simulink model "simplified_powertrain"  (R2020b)
settings: Solver=FixedStepAuto  StartTime=0.0  StopTime=60  RelTol=1e-3
PreLoadFcn:
  | C_sc = 1;
StartFcn:
  | C_sc = 1;
values from neighbouring files (symbols this model uses):
  D = 0    [model_fc.m]
undefined symbols (not defined in the file or in its folder): command, DiscIntNeverNeededParam, ECMS, Flight, in, Ion, Lithium, out, w
libraries: powerlib x22, electricdrivelib x3, lib_converters x3, simulink x2, fuzblock x1, mpclib x1, re_lib x1
(part 2 of 6)

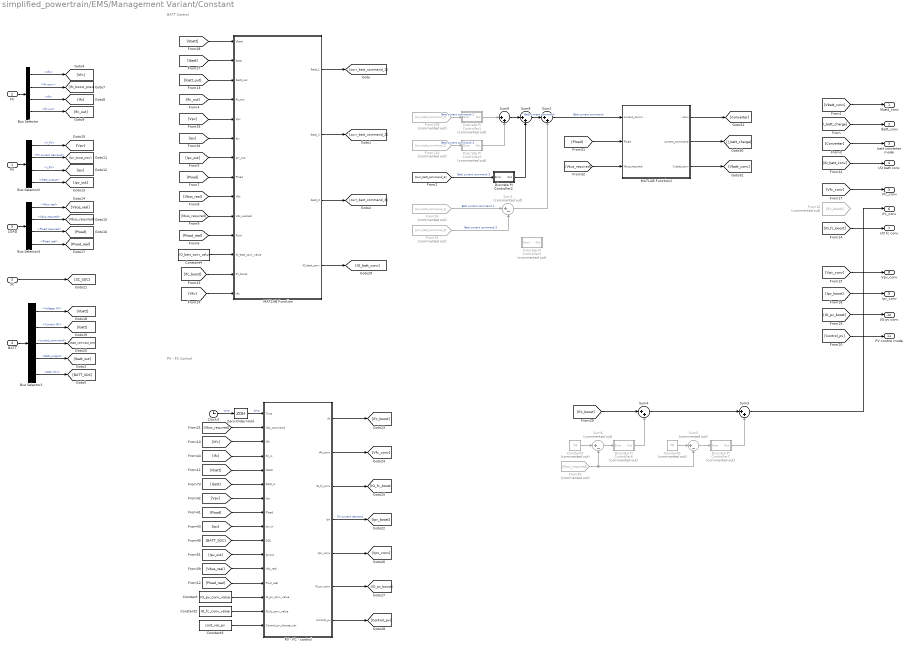
== system simplified_powertrain/EMS/Management Variant/Constant ==
  note: BATT Control
  note: PV - FC Control
  PV : Inport
  FC : Inport  Port=2
  SC : Inport  Port=3
  BATT : Inport  Port=4
  LOAD : Inport  Port=5
  Bus Selector : BusSelector  OutputSignals=Vfc,Ifc conv,Ifc,Ifc out
  Bus Selector1 : BusSelector  OutputSignals=Voltage (V),Current (A),current_command,Ibatt_output,SOC (%)
  Bus Selector2 : BusSelector  OutputSignals=V_PV,PV current demand,I_PV,Ibatt_output
  Bus Selector3 : BusSelector  OutputSignals=Vbus real,Vbus required,Pload required,Pload real
  Clock3 : Clock
  Constant : Constant  Value=IO_pv_conv_value
  Constant2 : Constant  Value=IO_fc_conv_value
  Constant3 : Constant  Value=cont_var_pv
  Constant4 : Constant  Value=IO_batt_conv_value
  Constant5 : Constant  Commented=on  Value=74
  Constant6 : Constant  Commented=on  Value=70
  Discrete PI Controller1 : Subsystem  Commented=on  DialogController=POWERSYS.PowerSysDialog  mask(Discrete PI Controller){Kp=1, Ki=10, Par_Limits=[100 -100], Init=0, Ts=1e-4}
      mask prompts: Kp "Proportional gain (Kp):"; Ki "Integral gain (Ki):"; Par_Limits "Output limits: [ Upper   Lower ]"; Init "Output initial value:"; Ts "Sample time:"
      mask help: This block implements a discrete PI controller.
      mask init:
      | UpperLimit=Par_Limits(1);
      | LowerLimit=Par_Limits(2);
      | power_initmask();
      mask Help: This block is part of a subset of blocks in the Extras library that does not have documentation associated with it, other than the block mask description.
      mask Display: disp('PI');
  Discrete PI Controller2 : Subsystem  DialogController=POWERSYS.PowerSysDialog  mask(Discrete PI Controller){Kp=10, Ki=100, Par_Limits=[100 -100], Init=0, Ts=1e-4}
      mask prompts: Kp "Proportional gain (Kp):"; Ki "Integral gain (Ki):"; Par_Limits "Output limits: [ Upper   Lower ]"; Init "Output initial value:"; Ts "Sample time:"
      mask help: This block implements a discrete PI controller.
      mask init:
      | UpperLimit=Par_Limits(1);
      | LowerLimit=Par_Limits(2);
      | power_initmask();
      mask Help: This block is part of a subset of blocks in the Extras library that does not have documentation associated with it, other than the block mask description.
      mask Display: disp('PI');
  Discrete PI Controller3 : Subsystem  Commented=on  DialogController=POWERSYS.PowerSysDialog  mask(Discrete PI Controller){Kp=10, Ki=1, Par_Limits=[100 -100], Init=0, Ts=1e-4}
      mask prompts: Kp "Proportional gain (Kp):"; Ki "Integral gain (Ki):"; Par_Limits "Output limits: [ Upper   Lower ]"; Init "Output initial value:"; Ts "Sample time:"
      mask help: This block implements a discrete PI controller.
      mask init:
      | UpperLimit=Par_Limits(1);
      | LowerLimit=Par_Limits(2);
      | power_initmask();
      mask Help: This block is part of a subset of blocks in the Extras library that does not have documentation associated with it, other than the block mask description.
      mask Display: disp('PI');
  Discrete PI Controller5 : Subsystem  Commented=on  DialogController=POWERSYS.PowerSysDialog  mask(Discrete PI Controller){Kp=10, Ki=10, Par_Limits=[50 -20], Init=0, Ts=1e-4}
      mask prompts: Kp "Proportional gain (Kp):"; Ki "Integral gain (Ki):"; Par_Limits "Output limits: [ Upper   Lower ]"; Init "Output initial value:"; Ts "Sample time:"
      mask help: This block implements a discrete PI controller.
      mask init:
      | UpperLimit=Par_Limits(1);
      | LowerLimit=Par_Limits(2);
      | power_initmask();
      mask Help: This block is part of a subset of blocks in the Extras library that does not have documentation associated with it, other than the block mask description.
      mask Display: disp('PI');
  Discrete PI Controller6 : Subsystem  Commented=on  DialogController=POWERSYS.PowerSysDialog  mask(Discrete PI Controller){Kp=10, Ki=10, Par_Limits=[40 0], Init=0, Ts=1e-4}
      mask prompts: Kp "Proportional gain (Kp):"; Ki "Integral gain (Ki):"; Par_Limits "Output limits: [ Upper   Lower ]"; Init "Output initial value:"; Ts "Sample time:"
      mask help: This block implements a discrete PI controller.
      mask init:
      | UpperLimit=Par_Limits(1);
      | LowerLimit=Par_Limits(2);
      | power_initmask();
      mask Help: This block is part of a subset of blocks in the Extras library that does not have documentation associated with it, other than the block mask description.
      mask Display: disp('PI');
  Discrete PI Controller7 : Subsystem  Commented=on  DialogController=POWERSYS.PowerSysDialog  mask(Discrete PI Controller){Kp=10, Ki=10, Par_Limits=[0 -40], Init=0, Ts=1e-4}
      mask prompts: Kp "Proportional gain (Kp):"; Ki "Integral gain (Ki):"; Par_Limits "Output limits: [ Upper   Lower ]"; Init "Output initial value:"; Ts "Sample time:"
      mask help: This block implements a discrete PI controller.
      mask init:
      | UpperLimit=Par_Limits(1);
      | LowerLimit=Par_Limits(2);
      | power_initmask();
      mask Help: This block is part of a subset of blocks in the Extras library that does not have documentation associated with it, other than the block mask description.
      mask Display: disp('PI');
  From108 : From  Commented=on  GotoTag=curr_batt_command_1
  From110 : From  Commented=on  GotoTag=curr_batt_command_2
  From16 : From  Commented=on  GotoTag=Ifc_boost
  From25 : From  Commented=on  GotoTag=curr_batt_command_3
  From26 : From  Commented=on  GotoTag=curr_batt_command_1
  From30 : From  Commented=on  GotoTag=Vbus_required
  MATLAB Function : MATLAB Function  TreatAsAtomicUnit=on
  MATLAB Function1 : MATLAB Function  TreatAsAtomicUnit=on
  PV - FC - control : MATLAB Function  TreatAsAtomicUnit=on
  Sum1 : Sum  Commented=on  Inputs=|+-
  Sum{2..4,8..9} (5 alike) : Sum  Inputs=|++
  Sum5 : Sum  Commented=on  Inputs=|+-
  Sum6 : Sum  Commented=on  Inputs=|+-
  Zero-Order Hold : ZeroOrderHold  SampleTime=1e-4
  Vbatt_conv : Outport
  Ibatt_conv : Outport  Port=2
  batt converter mode : Outport  Port=3
  I/O batt conv : Outport  Port=4
  Vfc_conv : Outport  Port=5
  Ifc_conv : Outport  Port=6
  I/O fc conv : Outport  Port=7
  Vpv_conv : Outport  Port=8
  Ipv_conv : Outport  Port=9
  I/O pv conv : Outport  Port=10
  PV control mode : Outport  Port=11
  wires:
  Constant/1 -> PV - FC - control/14(IO_pv_conv_value)
  MATLAB Function1/1(conv) -> [Converter]
  [Vbatt] -> MATLAB Function/1(Vbatt)
  [Ibatt_out] -> MATLAB Function/3(Ibatt_out)
  Bus Selector1/5 -> [BATT_SOC]  "<SOC (%)>"
  From30/1 -> Sum5/2, Sum6/2
  [Vpv] -> MATLAB Function/5(Vpv)
  Sum6/1 -> Discrete PI Controller6/1(Error)
  Discrete PI Controller7/1(Out) -> Sum3/2
  PV - FC - control/3(IO_fc_conv) -> [IO_fc_boost]
  [Ifc_out] -> MATLAB Function/4(Ifc_out)
  Bus Selector1/3 -> [Ibatt_command_pre]  "<current_command>"
  [IO_fc_boost] -> I/O fc conv/1
  MATLAB Function1/3(V_batt_conv) -> [Vbatt_conv]
  Bus Selector1/2 -> [Ibatt]  "<Current (A)>"
  [Ifc_boost] -> MATLAB Function/13(Ifc_boost)
  [Vbus_required] -> MATLAB Function1/3(Vbus_required)
  Sum2/1 -> MATLAB Function1/1(current_comm)  "Batt current command"
  [Vpv_conv] -> Vpv_conv/1
  Bus Selector1/1 -> [Vbatt]  "<Voltage (V)>"
  [Ibatt] -> PV - FC - control/6(Ibatt_in)
  From26/1 -> Sum1/1  "Batt current command 1"
  Bus Selector1/4 -> [Ibatt_out]  "<Ibatt_output>"
  MATLAB Function1/2(current_command) -> [I_batt_charge]
  [Ipv_boost] -> Ipv_conv/1
  [Pload_real] -> MATLAB Function/11(Pout)
  PV - FC - control/5(Vpv_conv) -> [Vpv_conv]
  Constant6/1 -> Sum5/1
  Sum5/1 -> Discrete PI Controller7/1(Error)
  Constant2/1 -> PV - FC - control/15(IO_fc_conv_value)
  MATLAB Function/2(Ibatt_2) -> [curr_batt_command_2]
  MATLAB Function/1(Ibatt_1) -> [curr_batt_command_1]
  Bus Selector2/1 -> [Vpv]  "<V_PV>"
  [Pload] -> MATLAB Function1/2(Pload)
  Sum4/1 -> Sum3/1
  [Ifc_boost] -> Sum4/1
  From25/1 -> Sum1/2  "Batt current command 3"
  [Ibatt] -> MATLAB Function/2(Ibatt)
  [IO_pv_boost] -> I/O pv conv/1
  [Vfc] -> MATLAB Function/14(Vfc)
  Bus Selector2/3 -> [Ipv]  "<I_PV>"
  Sum1/1 -> Sum2/2
  [Vfc_conv] -> Vfc_conv/1
  [Ipv_out] -> PV - FC - control/11(Ipvout)
  PV - FC - control/7(Control_pv) -> [Control_pv]
  [Vbus_required] -> PV - FC - control/2(Vdc_command)
  [Vbatt_conv] -> Vbatt_conv/1
  [Vbus_real] -> PV - FC - control/12(Vdc_real)
  MATLAB Function/4(IO_batt_conv) -> [IO_batt_conv]
  Constant3/1 -> PV - FC - control/16(Control_pv_choose_var)
  PV - FC - control/1(Ifc) -> [Ifc_boost]
  FC/1 -> Bus Selector/1
  [Ipv] -> PV - FC - control/9(Ipv_in)
  Sum8/1 -> Sum2/1  "Batt current command"
  Zero-Order Hold/1 -> PV - FC - control/1(Time)  "time"
  [Pload] -> MATLAB Function/8(Pload)
  [Vbus_required] -> MATLAB Function/10(Vdc_wanted)
  Clock3/1 -> Zero-Order Hold/1  "time"
  [Pload_real] -> PV - FC - control/13(Pout_real)
  [Vpv] -> PV - FC - control/7(Vpv)
  LOAD/1 -> Bus Selector3/1
  Constant5/1 -> Sum6/1
  [Control_pv] -> PV control mode/1
  Bus Selector/3 -> [Ifc]  "<Ifc>"
  [Ipv_out] -> MATLAB Function/7(Ipv_out)
  From110/1 -> Discrete PI Controller3/1(Error)  "Batt current command 3"
  [IO_batt_conv] -> I/O batt conv/1
  [Vbus_real] -> MATLAB Function/9(Vdc)
  Bus Selector3/3 -> [Pload]  "<Pload required>"
  Bus Selector2/4 -> [Ipv_out]  "<Ibatt_output>"
  PV - FC - control/4(Ipv) -> [Ipv_boost]  "PV current demand"
  [Ifc] -> PV - FC - control/4(Ifc_in)
  Bus Selector3/2 -> [Vbus_required]  "<Vbus required>"
  BATT/1 -> Bus Selector1/1
  Discrete PI Controller6/1(Out) -> Sum4/2
  Bus Selector2/2 -> [Ipv_boost_prev]  "<PV current demand>"
  Bus Selector3/1 -> [Vbus_real]  "<Vbus real>"
  Constant4/1 -> MATLAB Function/12(IO_batt_conv_value)
  PV - FC - control/6(IO_pv_conv) -> [IO_pv_boost]
  SC/1 -> [SC_SOC]
  [Converter] -> batt converter mode/1
  PV - FC - control/2(Vfc_conv) -> [Vfc_conv]
  [I_batt_charge] -> Ibatt_conv/1
  [Vbatt] -> PV - FC - control/5(Vbatt)
  [Vfc] -> PV - FC - control/3(Vfc)
  [curr_batt_command_3] -> Discrete PI Controller2/1(Error)  "Batt current command 3"
  Bus Selector/1 -> [Vfc]  "<Vfc>"
  Bus Selector/4 -> [Ifc_out]  "<Ifc out>"
  PV/1 -> Bus Selector2/1
  [Pload] -> PV - FC - control/8(Pload)
  Bus Selector/2 -> [Ifc_boost_prev]  "<Ifc conv>"
  Sum9/1 -> Sum8/1
  From108/1 -> Discrete PI Controller1/1(Error)  "Batt current command 1"
  Discrete PI Controller2/1(Out) -> Sum8/2
  MATLAB Function/3(Ibatt_3) -> [curr_batt_command_3]
  Sum3/1 -> Ifc_conv/1
  Discrete PI Controller1/1(Out) -> Sum9/1
  Discrete PI Controller3/1(Out) -> Sum9/2
  [BATT_SOC] -> PV - FC - control/10(SOC)
  [Ipv] -> MATLAB Function/6(Ipv)
  Bus Selector3/4 -> [Pload_real]  "<Pload real>"

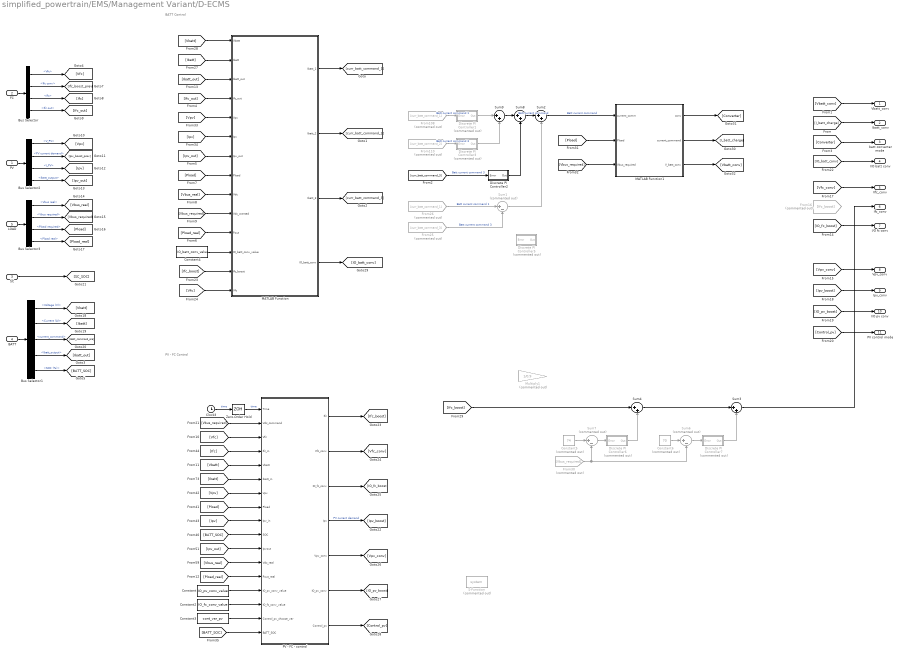
== system simplified_powertrain/EMS/Management Variant/D-ECMS ==
  note: PV - FC Control
  note: BATT Control
  PV : Inport
  FC : Inport  Port=2
  SC : Inport  Port=3
  BATT : Inport  Port=4
  LOAD : Inport  Port=5
  Bus Selector : BusSelector  OutputSignals=Vfc,Ifc conv,Ifc,Ifc out
  Bus Selector1 : BusSelector  OutputSignals=Voltage (V),Current (A),current_command,Ibatt_output,SOC (%)
  Bus Selector2 : BusSelector  OutputSignals=V_PV,PV current demand,I_PV,Ibatt_output
  Bus Selector3 : BusSelector  OutputSignals=Vbus real,Vbus required,Pload required,Pload real
  Clock3 : Clock
  Constant : Constant  Value=IO_pv_conv_value
  Constant2 : Constant  Value=IO_fc_conv_value
  Constant3 : Constant  Value=cont_var_pv
  Constant4 : Constant  Value=IO_batt_conv_value
  Constant5 : Constant  Commented=on  Value=74
  Constant6 : Constant  Commented=on  Value=70
  Discrete PI Controller1 : Subsystem  Commented=on  DialogController=POWERSYS.PowerSysDialog  mask(Discrete PI Controller){Kp=1, Ki=10, Par_Limits=[100 -100], Init=0, Ts=1e-4}
      mask prompts: Kp "Proportional gain (Kp):"; Ki "Integral gain (Ki):"; Par_Limits "Output limits: [ Upper   Lower ]"; Init "Output initial value:"; Ts "Sample time:"
      mask help: This block implements a discrete PI controller.
      mask init:
      | UpperLimit=Par_Limits(1);
      | LowerLimit=Par_Limits(2);
      | power_initmask();
      mask Help: This block is part of a subset of blocks in the Extras library that does not have documentation associated with it, other than the block mask description.
      mask Display: disp('PI');
  Discrete PI Controller2 : Subsystem  DialogController=POWERSYS.PowerSysDialog  mask(Discrete PI Controller){Kp=10, Ki=100, Par_Limits=[50 -20], Init=0, Ts=1e-4}
      mask prompts: Kp "Proportional gain (Kp):"; Ki "Integral gain (Ki):"; Par_Limits "Output limits: [ Upper   Lower ]"; Init "Output initial value:"; Ts "Sample time:"
      mask help: This block implements a discrete PI controller.
      mask init:
      | UpperLimit=Par_Limits(1);
      | LowerLimit=Par_Limits(2);
      | power_initmask();
      mask Help: This block is part of a subset of blocks in the Extras library that does not have documentation associated with it, other than the block mask description.
      mask Display: disp('PI');
  Discrete PI Controller3 : Subsystem  Commented=on  DialogController=POWERSYS.PowerSysDialog  mask(Discrete PI Controller){Kp=10, Ki=1, Par_Limits=[100 -100], Init=0, Ts=1e-4}
      mask prompts: Kp "Proportional gain (Kp):"; Ki "Integral gain (Ki):"; Par_Limits "Output limits: [ Upper   Lower ]"; Init "Output initial value:"; Ts "Sample time:"
      mask help: This block implements a discrete PI controller.
      mask init:
      | UpperLimit=Par_Limits(1);
      | LowerLimit=Par_Limits(2);
      | power_initmask();
      mask Help: This block is part of a subset of blocks in the Extras library that does not have documentation associated with it, other than the block mask description.
      mask Display: disp('PI');
  Discrete PI Controller5 : Subsystem  Commented=on  DialogController=POWERSYS.PowerSysDialog  mask(Discrete PI Controller){Kp=10, Ki=10, Par_Limits=[50 -20], Init=0, Ts=1e-4}
      mask prompts: Kp "Proportional gain (Kp):"; Ki "Integral gain (Ki):"; Par_Limits "Output limits: [ Upper   Lower ]"; Init "Output initial value:"; Ts "Sample time:"
      mask help: This block implements a discrete PI controller.
      mask init:
      | UpperLimit=Par_Limits(1);
      | LowerLimit=Par_Limits(2);
      | power_initmask();
      mask Help: This block is part of a subset of blocks in the Extras library that does not have documentation associated with it, other than the block mask description.
      mask Display: disp('PI');
  Discrete PI Controller6 : Subsystem  Commented=on  DialogController=POWERSYS.PowerSysDialog  mask(Discrete PI Controller){Kp=10, Ki=10, Par_Limits=[40 0], Init=0, Ts=1e-4}
      mask prompts: Kp "Proportional gain (Kp):"; Ki "Integral gain (Ki):"; Par_Limits "Output limits: [ Upper   Lower ]"; Init "Output initial value:"; Ts "Sample time:"
      mask help: This block implements a discrete PI controller.
      mask init:
      | UpperLimit=Par_Limits(1);
      | LowerLimit=Par_Limits(2);
      | power_initmask();
      mask Help: This block is part of a subset of blocks in the Extras library that does not have documentation associated with it, other than the block mask description.
      mask Display: disp('PI');
  Discrete PI Controller7 : Subsystem  Commented=on  DialogController=POWERSYS.PowerSysDialog  mask(Discrete PI Controller){Kp=10, Ki=10, Par_Limits=[0 -40], Init=0, Ts=1e-4}
      mask prompts: Kp "Proportional gain (Kp):"; Ki "Integral gain (Ki):"; Par_Limits "Output limits: [ Upper   Lower ]"; Init "Output initial value:"; Ts "Sample time:"
      mask help: This block implements a discrete PI controller.
      mask init:
      | UpperLimit=Par_Limits(1);
      | LowerLimit=Par_Limits(2);
      | power_initmask();
      mask Help: This block is part of a subset of blocks in the Extras library that does not have documentation associated with it, other than the block mask description.
      mask Display: disp('PI');
  From108 : From  Commented=on  GotoTag=curr_batt_command_1
  From110 : From  Commented=on  GotoTag=curr_batt_command_2
  From16 : From  Commented=on  GotoTag=Ifc_boost
  From25 : From  Commented=on  GotoTag=curr_batt_command_3
  From26 : From  Commented=on  GotoTag=curr_batt_command_1
  From30 : From  Commented=on  GotoTag=Vbus_required
  MATLAB Function : MATLAB Function  TreatAsAtomicUnit=on
  MATLAB Function1 : MATLAB Function  TreatAsAtomicUnit=on
  Multiply1 : Gain  Commented=on  Gain=1/0.9
  PV - FC - control : MATLAB Function  TreatAsAtomicUnit=on
  S-Function : S-Function  Commented=on  SFunctionDeploymentMode=off  EnableBusSupport=off
  Sum1 : Sum  Commented=on  Inputs=|+-
  Sum{2..4,8..9} (5 alike) : Sum  Inputs=|++
  Sum6 : Sum  Commented=on  Inputs=|+-
  Sum7 : Sum  Commented=on  Inputs=|+-
  Zero-Order Hold : ZeroOrderHold  SampleTime=1e-4
  Vbatt_conv : Outport
  Ibatt_conv : Outport  Port=2
  batt converter mode : Outport  Port=3
  I/O batt conv : Outport  Port=4
  Vfc_conv : Outport  Port=5
  Ifc_conv : Outport  Port=6
  I/O fc conv : Outport  Port=7
  Vpv_conv : Outport  Port=8
  Ipv_conv : Outport  Port=9
  I/O pv conv : Outport  Port=10
  PV control mode : Outport  Port=11
  wires:
  [Ipv_out] -> PV - FC - control/11(Ipvout)
  Sum1/1 -> Sum2/2
  PV - FC - control/7(Control_pv) -> [Control_pv]
  [Vbus_required] -> PV - FC - control/2(Vdc_command)
  MATLAB Function/4(IO_batt_conv) -> [IO_batt_conv]
  Constant3/1 -> PV - FC - control/16(Control_pv_choose_var)
  [Vbatt_conv] -> Vbatt_conv/1
  [Vbus_real] -> PV - FC - control/12(Vdc_real)
  [Pload] -> MATLAB Function/8(Pload)
  Zero-Order Hold/1 -> PV - FC - control/1(Time)  "time"
  [Ipv] -> PV - FC - control/9(Ipv_in)
  Sum8/1 -> Sum2/1  "Batt current command"
  [Vpv] -> PV - FC - control/7(Vpv)
  LOAD/1 -> Bus Selector3/1
  Clock3/1 -> Zero-Order Hold/1  "time"
  [Control_pv] -> PV control mode/1
  [Ipv_out] -> MATLAB Function/7(Ipv_out)
  Bus Selector/3 -> [Ifc]  "<Ifc>"
  [IO_batt_conv] -> I/O batt conv/1
  Bus Selector3/3 -> [Pload]  "<Pload required>"
  PV - FC - control/4(Ipv) -> [Ipv_boost]  "PV current demand"
  Bus Selector2/4 -> [Ipv_out]  "<Ibatt_output>"
  [Ifc_boost] -> Sum4/1
  [Vbus_required] -> MATLAB Function/10(Vdc_wanted)
  [BATT_SOC] -> PV - FC - control/17(BATT_SOC)
  PV/1 -> Bus Selector2/1
  [curr_batt_command_3] -> Discrete PI Controller2/1(Error)  "Batt current command 3"
  From110/1 -> Discrete PI Controller3/1(Error)  "Batt current command 3"
  [Vbus_required] -> MATLAB Function1/3(Vbus_required)
  Bus Selector1/3 -> [Ibatt_command_pre]  "<current_command>"
  PV - FC - control/3(IO_fc_conv) -> [IO_fc_boost]
  [Ifc_out] -> MATLAB Function/4(Ifc_out)
  [Vpv_conv] -> Vpv_conv/1
  Bus Selector1/2 -> [Ibatt]  "<Current (A)>"
  MATLAB Function1/3(V_batt_conv) -> [Vbatt_conv]
  [Ifc_boost] -> MATLAB Function/13(Ifc_boost)
  Bus Selector/2 -> [Ifc_boost_prev]  "<Ifc conv>"
  Bus Selector3/4 -> [Pload_real]  "<Pload real>"
  Discrete PI Controller3/1(Out) -> Sum9/2
  [Ifc] -> PV - FC - control/4(Ifc_in)
  Discrete PI Controller6/1(Out) -> Sum4/2
  [Vbatt] -> MATLAB Function/1(Vbatt)
  PV - FC - control/6(IO_pv_conv) -> [IO_pv_boost]
  Discrete PI Controller2/1(Out) -> Sum8/2
  Bus Selector1/5 -> [BATT_SOC]  "<SOC (%)>"
  Bus Selector1/4 -> [Ibatt_out]  "<Ibatt_output>"
  [Vbatt] -> PV - FC - control/5(Vbatt)
  [Ipv_boost] -> Ipv_conv/1
  Sum7/1 -> Discrete PI Controller6/1(Error)
  Bus Selector3/2 -> [Vbus_required]  "<Vbus required>"
  Bus Selector3/1 -> [Vbus_real]  "<Vbus real>"
  Bus Selector2/2 -> [Ipv_boost_prev]  "<PV current demand>"
  FC/1 -> Bus Selector/1
  PV - FC - control/2(Vfc_conv) -> [Vfc_conv]
  Bus Selector/4 -> [Ifc_out]  "<Ifc out>"
  PV - FC - control/1(Ifc) -> [Ifc_boost]
  [BATT_SOC] -> PV - FC - control/10(SOC)
  [Vfc] -> PV - FC - control/3(Vfc)
  [Pload] -> PV - FC - control/8(Pload)
  Sum6/1 -> Discrete PI Controller7/1(Error)
  From26/1 -> Sum1/1  "Batt current command 1"
  [Pload_real] -> MATLAB Function/11(Pout)
  PV - FC - control/5(Vpv_conv) -> [Vpv_conv]
  MATLAB Function1/2(current_command) -> [I_batt_charge]
  [Ibatt_out] -> MATLAB Function/3(Ibatt_out)
  Constant6/1 -> Sum6/1
  Sum4/1 -> Sum3/1
  SC/1 -> [SC_SOC]
  [Ipv] -> MATLAB Function/6(Ipv)
  Bus Selector2/1 -> [Vpv]  "<V_PV>"
  Constant2/1 -> PV - FC - control/15(IO_fc_conv_value)
  [Pload] -> MATLAB Function1/2(Pload)
  MATLAB Function/1(Ibatt_1) -> [curr_batt_command_1]
  Constant5/1 -> Sum7/1
  Constant4/1 -> MATLAB Function/12(IO_batt_conv_value)
  MATLAB Function/2(Ibatt_2) -> [curr_batt_command_2]
  [IO_fc_boost] -> I/O fc conv/1
  [Ibatt] -> MATLAB Function/2(Ibatt)
  From108/1 -> Discrete PI Controller1/1(Error)  "Batt current command 1"
  [IO_pv_boost] -> I/O pv conv/1
  Bus Selector2/3 -> [Ipv]  "<I_PV>"
  [Vfc] -> MATLAB Function/14(Vfc)
  MATLAB Function/3(Ibatt_3) -> [curr_batt_command_3]
  From25/1 -> Sum1/2  "Batt current command 3"
  BATT/1 -> Bus Selector1/1
  Sum3/1 -> Ifc_conv/1
  [Vfc_conv] -> Vfc_conv/1
  Sum2/1 -> MATLAB Function1/1(current_comm)  "Batt current command"
  Bus Selector/1 -> [Vfc]  "<Vfc>"
  [Pload_real] -> PV - FC - control/13(Pout_real)
  [Ibatt] -> PV - FC - control/6(Ibatt_in)
  [Vpv] -> MATLAB Function/5(Vpv)
  [Vbus_real] -> MATLAB Function/9(Vdc)
  Discrete PI Controller7/1(Out) -> Sum3/2
  Bus Selector1/1 -> [Vbatt]  "<Voltage (V)>"
  Sum9/1 -> Sum8/1
  [Converter] -> batt converter mode/1
  MATLAB Function1/1(conv) -> [Converter]
  Constant/1 -> PV - FC - control/14(IO_pv_conv_value)
  [I_batt_charge] -> Ibatt_conv/1
  From30/1 -> Sum6/2, Sum7/2
  Discrete PI Controller1/1(Out) -> Sum9/1

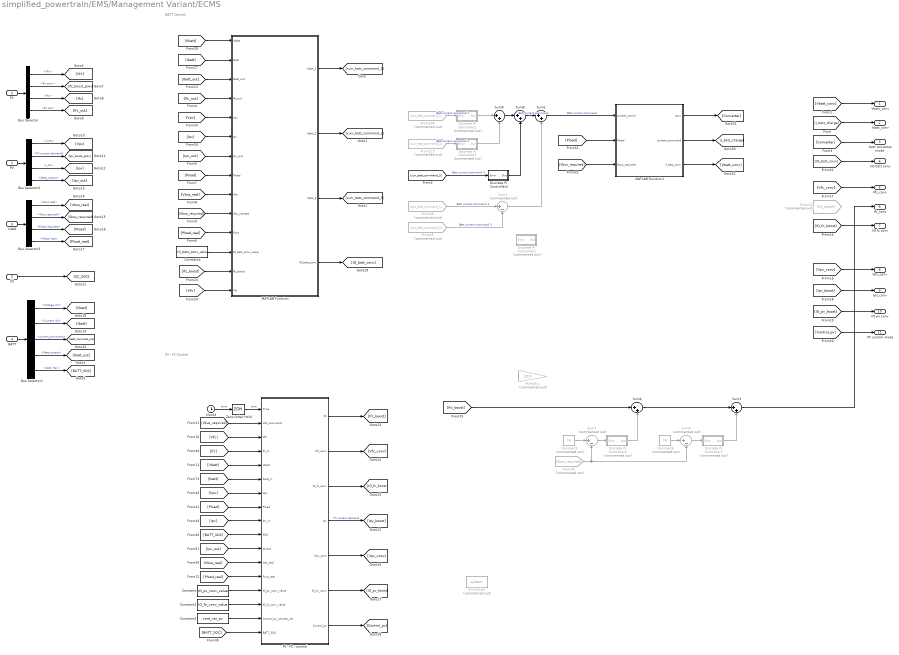
== system simplified_powertrain/EMS/Management Variant/ECMS ==
  note: PV - FC Control
  note: BATT Control
  PV : Inport
  FC : Inport  Port=2
  SC : Inport  Port=3
  BATT : Inport  Port=4
  LOAD : Inport  Port=5
  Bus Selector : BusSelector  OutputSignals=Vfc,Ifc conv,Ifc,Ifc out
  Bus Selector1 : BusSelector  OutputSignals=Voltage (V),Current (A),current_command,Ibatt_output,SOC (%)
  Bus Selector2 : BusSelector  OutputSignals=V_PV,PV current demand,I_PV,Ibatt_output
  Bus Selector3 : BusSelector  OutputSignals=Vbus real,Vbus required,Pload required,Pload real
  Clock3 : Clock
  Constant : Constant  Value=IO_pv_conv_value
  Constant2 : Constant  Value=IO_fc_conv_value
  Constant3 : Constant  Value=cont_var_pv
  Constant4 : Constant  Value=IO_batt_conv_value
  Constant5 : Constant  Commented=on  Value=74
  Constant6 : Constant  Commented=on  Value=70
  Discrete PI Controller1 : Subsystem  Commented=on  DialogController=POWERSYS.PowerSysDialog  mask(Discrete PI Controller){Kp=1, Ki=10, Par_Limits=[100 -100], Init=0, Ts=1e-4}
      mask prompts: Kp "Proportional gain (Kp):"; Ki "Integral gain (Ki):"; Par_Limits "Output limits: [ Upper   Lower ]"; Init "Output initial value:"; Ts "Sample time:"
      mask help: This block implements a discrete PI controller.
      mask init:
      | UpperLimit=Par_Limits(1);
      | LowerLimit=Par_Limits(2);
      | power_initmask();
      mask Help: This block is part of a subset of blocks in the Extras library that does not have documentation associated with it, other than the block mask description.
      mask Display: disp('PI');
  Discrete PI Controller2 : Subsystem  DialogController=POWERSYS.PowerSysDialog  mask(Discrete PI Controller){Kp=10, Ki=100, Par_Limits=[50 -20], Init=0, Ts=1e-4}
      mask prompts: Kp "Proportional gain (Kp):"; Ki "Integral gain (Ki):"; Par_Limits "Output limits: [ Upper   Lower ]"; Init "Output initial value:"; Ts "Sample time:"
      mask help: This block implements a discrete PI controller.
      mask init:
      | UpperLimit=Par_Limits(1);
      | LowerLimit=Par_Limits(2);
      | power_initmask();
      mask Help: This block is part of a subset of blocks in the Extras library that does not have documentation associated with it, other than the block mask description.
      mask Display: disp('PI');
  Discrete PI Controller3 : Subsystem  Commented=on  DialogController=POWERSYS.PowerSysDialog  mask(Discrete PI Controller){Kp=10, Ki=1, Par_Limits=[100 -100], Init=0, Ts=1e-4}
      mask prompts: Kp "Proportional gain (Kp):"; Ki "Integral gain (Ki):"; Par_Limits "Output limits: [ Upper   Lower ]"; Init "Output initial value:"; Ts "Sample time:"
      mask help: This block implements a discrete PI controller.
      mask init:
      | UpperLimit=Par_Limits(1);
      | LowerLimit=Par_Limits(2);
      | power_initmask();
      mask Help: This block is part of a subset of blocks in the Extras library that does not have documentation associated with it, other than the block mask description.
      mask Display: disp('PI');
  Discrete PI Controller5 : Subsystem  Commented=on  DialogController=POWERSYS.PowerSysDialog  mask(Discrete PI Controller){Kp=10, Ki=10, Par_Limits=[50 -20], Init=0, Ts=1e-4}
      mask prompts: Kp "Proportional gain (Kp):"; Ki "Integral gain (Ki):"; Par_Limits "Output limits: [ Upper   Lower ]"; Init "Output initial value:"; Ts "Sample time:"
      mask help: This block implements a discrete PI controller.
      mask init:
      | UpperLimit=Par_Limits(1);
      | LowerLimit=Par_Limits(2);
      | power_initmask();
      mask Help: This block is part of a subset of blocks in the Extras library that does not have documentation associated with it, other than the block mask description.
      mask Display: disp('PI');
  Discrete PI Controller6 : Subsystem  Commented=on  DialogController=POWERSYS.PowerSysDialog  mask(Discrete PI Controller){Kp=10, Ki=10, Par_Limits=[40 0], Init=0, Ts=1e-4}
      mask prompts: Kp "Proportional gain (Kp):"; Ki "Integral gain (Ki):"; Par_Limits "Output limits: [ Upper   Lower ]"; Init "Output initial value:"; Ts "Sample time:"
      mask help: This block implements a discrete PI controller.
      mask init:
      | UpperLimit=Par_Limits(1);
      | LowerLimit=Par_Limits(2);
      | power_initmask();
      mask Help: This block is part of a subset of blocks in the Extras library that does not have documentation associated with it, other than the block mask description.
      mask Display: disp('PI');
  Discrete PI Controller7 : Subsystem  Commented=on  DialogController=POWERSYS.PowerSysDialog  mask(Discrete PI Controller){Kp=10, Ki=10, Par_Limits=[0 -40], Init=0, Ts=1e-4}
      mask prompts: Kp "Proportional gain (Kp):"; Ki "Integral gain (Ki):"; Par_Limits "Output limits: [ Upper   Lower ]"; Init "Output initial value:"; Ts "Sample time:"
      mask help: This block implements a discrete PI controller.
      mask init:
      | UpperLimit=Par_Limits(1);
      | LowerLimit=Par_Limits(2);
      | power_initmask();
      mask Help: This block is part of a subset of blocks in the Extras library that does not have documentation associated with it, other than the block mask description.
      mask Display: disp('PI');
  From108 : From  Commented=on  GotoTag=curr_batt_command_1
  From110 : From  Commented=on  GotoTag=curr_batt_command_2
  From16 : From  Commented=on  GotoTag=Ifc_boost
  From25 : From  Commented=on  GotoTag=curr_batt_command_3
  From26 : From  Commented=on  GotoTag=curr_batt_command_1
  From30 : From  Commented=on  GotoTag=Vbus_required
  MATLAB Function : MATLAB Function  TreatAsAtomicUnit=on
  MATLAB Function1 : MATLAB Function  TreatAsAtomicUnit=on
  Multiply1 : Gain  Commented=on  Gain=1/0.9
  PV - FC - control : MATLAB Function  TreatAsAtomicUnit=on
  S-Function : S-Function  Commented=on  SFunctionDeploymentMode=off  EnableBusSupport=off
  Sum1 : Sum  Commented=on  Inputs=|+-
  Sum{2..4,8..9} (5 alike) : Sum  Inputs=|++
  Sum6 : Sum  Commented=on  Inputs=|+-
  Sum7 : Sum  Commented=on  Inputs=|+-
  Zero-Order Hold : ZeroOrderHold  SampleTime=1e-4
  Vbatt_conv : Outport
  Ibatt_conv : Outport  Port=2
  batt converter mode : Outport  Port=3
  I/O batt conv : Outport  Port=4
  Vfc_conv : Outport  Port=5
  Ifc_conv : Outport  Port=6
  I/O fc conv : Outport  Port=7
  Vpv_conv : Outport  Port=8
  Ipv_conv : Outport  Port=9
  I/O pv conv : Outport  Port=10
  PV control mode : Outport  Port=11
  wires:
  [Ipv_out] -> PV - FC - control/11(Ipvout)
  Sum1/1 -> Sum2/2
  PV - FC - control/7(Control_pv) -> [Control_pv]
  [Vbus_required] -> PV - FC - control/2(Vdc_command)
  MATLAB Function/4(IO_batt_conv) -> [IO_batt_conv]
  Constant3/1 -> PV - FC - control/16(Control_pv_choose_var)
  [Vbatt_conv] -> Vbatt_conv/1
  [Vbus_real] -> PV - FC - control/12(Vdc_real)
  [Pload] -> MATLAB Function/8(Pload)
  Zero-Order Hold/1 -> PV - FC - control/1(Time)  "time"
  [Ipv] -> PV - FC - control/9(Ipv_in)
  Sum8/1 -> Sum2/1  "Batt current command"
  [Vpv] -> PV - FC - control/7(Vpv)
  LOAD/1 -> Bus Selector3/1
  Clock3/1 -> Zero-Order Hold/1  "time"
  [Control_pv] -> PV control mode/1
  [Ipv_out] -> MATLAB Function/7(Ipv_out)
  Bus Selector/3 -> [Ifc]  "<Ifc>"
  [IO_batt_conv] -> I/O batt conv/1
  Bus Selector3/3 -> [Pload]  "<Pload required>"
  PV - FC - control/4(Ipv) -> [Ipv_boost]  "PV current demand"
  Bus Selector2/4 -> [Ipv_out]  "<Ibatt_output>"
  [Ifc_boost] -> Sum4/1
  [Vbus_required] -> MATLAB Function/10(Vdc_wanted)
  [BATT_SOC] -> PV - FC - control/17(BATT_SOC)
  PV/1 -> Bus Selector2/1
  [curr_batt_command_3] -> Discrete PI Controller2/1(Error)  "Batt current command 3"
  From110/1 -> Discrete PI Controller3/1(Error)  "Batt current command 3"
  [Vbus_required] -> MATLAB Function1/3(Vbus_required)
  Bus Selector1/3 -> [Ibatt_command_pre]  "<current_command>"
  PV - FC - control/3(IO_fc_conv) -> [IO_fc_boost]
  [Ifc_out] -> MATLAB Function/4(Ifc_out)
  [Vpv_conv] -> Vpv_conv/1
  Bus Selector1/2 -> [Ibatt]  "<Current (A)>"
  MATLAB Function1/3(V_batt_conv) -> [Vbatt_conv]
  [Ifc_boost] -> MATLAB Function/13(Ifc_boost)
  Bus Selector/2 -> [Ifc_boost_prev]  "<Ifc conv>"
  Bus Selector3/4 -> [Pload_real]  "<Pload real>"
  Discrete PI Controller3/1(Out) -> Sum9/2
  [Ifc] -> PV - FC - control/4(Ifc_in)
  Discrete PI Controller6/1(Out) -> Sum4/2
  [Vbatt] -> MATLAB Function/1(Vbatt)
  PV - FC - control/6(IO_pv_conv) -> [IO_pv_boost]
  Discrete PI Controller2/1(Out) -> Sum8/2
  Bus Selector1/5 -> [BATT_SOC]  "<SOC (%)>"
  Bus Selector1/4 -> [Ibatt_out]  "<Ibatt_output>"
  [Vbatt] -> PV - FC - control/5(Vbatt)
  [Ipv_boost] -> Ipv_conv/1
  Sum7/1 -> Discrete PI Controller6/1(Error)
  Bus Selector3/2 -> [Vbus_required]  "<Vbus required>"
  Bus Selector3/1 -> [Vbus_real]  "<Vbus real>"
  Bus Selector2/2 -> [Ipv_boost_prev]  "<PV current demand>"
  FC/1 -> Bus Selector/1
  PV - FC - control/2(Vfc_conv) -> [Vfc_conv]
  Bus Selector/4 -> [Ifc_out]  "<Ifc out>"
  PV - FC - control/1(Ifc) -> [Ifc_boost]
  [BATT_SOC] -> PV - FC - control/10(SOC)
  [Vfc] -> PV - FC - control/3(Vfc)
  [Pload] -> PV - FC - control/8(Pload)
  Sum6/1 -> Discrete PI Controller7/1(Error)
  From26/1 -> Sum1/1  "Batt current command 1"
  [Pload_real] -> MATLAB Function/11(Pout)
  PV - FC - control/5(Vpv_conv) -> [Vpv_conv]
  MATLAB Function1/2(current_command) -> [I_batt_charge]
  [Ibatt_out] -> MATLAB Function/3(Ibatt_out)
  Constant6/1 -> Sum6/1
  Sum4/1 -> Sum3/1
  SC/1 -> [SC_SOC]
  [Ipv] -> MATLAB Function/6(Ipv)
  Bus Selector2/1 -> [Vpv]  "<V_PV>"
  Constant2/1 -> PV - FC - control/15(IO_fc_conv_value)
  [Pload] -> MATLAB Function1/2(Pload)
  MATLAB Function/1(Ibatt_1) -> [curr_batt_command_1]
  Constant5/1 -> Sum7/1
  Constant4/1 -> MATLAB Function/12(IO_batt_conv_value)
  MATLAB Function/2(Ibatt_2) -> [curr_batt_command_2]
  [IO_fc_boost] -> I/O fc conv/1
  [Ibatt] -> MATLAB Function/2(Ibatt)
  From108/1 -> Discrete PI Controller1/1(Error)  "Batt current command 1"
  [IO_pv_boost] -> I/O pv conv/1
  Bus Selector2/3 -> [Ipv]  "<I_PV>"
  [Vfc] -> MATLAB Function/14(Vfc)
  MATLAB Function/3(Ibatt_3) -> [curr_batt_command_3]
  From25/1 -> Sum1/2  "Batt current command 3"
  BATT/1 -> Bus Selector1/1
  Sum3/1 -> Ifc_conv/1
  [Vfc_conv] -> Vfc_conv/1
  Sum2/1 -> MATLAB Function1/1(current_comm)  "Batt current command"
  Bus Selector/1 -> [Vfc]  "<Vfc>"
  [Pload_real] -> PV - FC - control/13(Pout_real)
  [Ibatt] -> PV - FC - control/6(Ibatt_in)
  [Vpv] -> MATLAB Function/5(Vpv)
  [Vbus_real] -> MATLAB Function/9(Vdc)
  Discrete PI Controller7/1(Out) -> Sum3/2
  Bus Selector1/1 -> [Vbatt]  "<Voltage (V)>"
  Sum9/1 -> Sum8/1
  [Converter] -> batt converter mode/1
  MATLAB Function1/1(conv) -> [Converter]
  Constant/1 -> PV - FC - control/14(IO_pv_conv_value)
  [I_batt_charge] -> Ibatt_conv/1
  From30/1 -> Sum6/2, Sum7/2
  Discrete PI Controller1/1(Out) -> Sum9/1

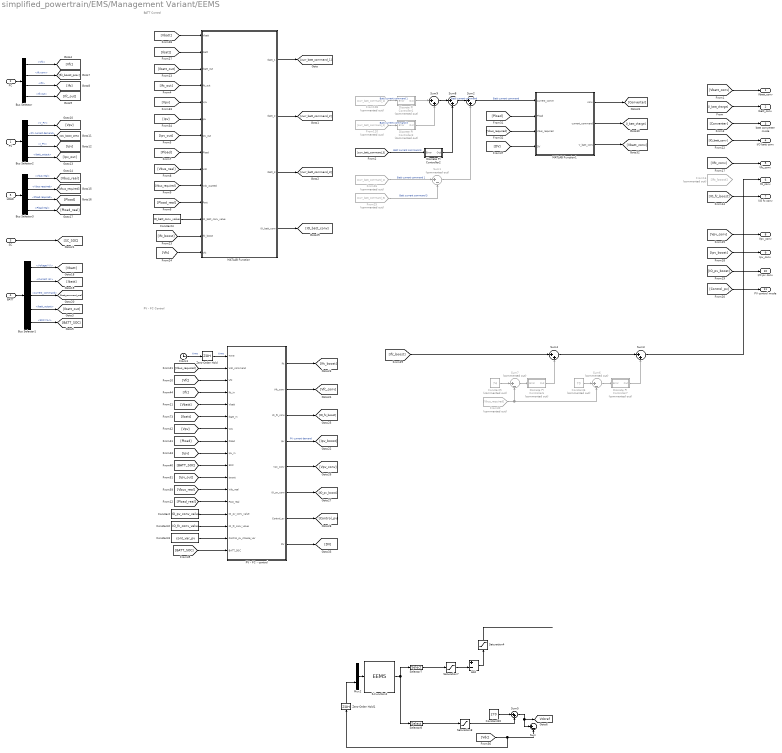
== system simplified_powertrain/EMS/Management Variant/EEMS ==
  note: PV - FC Control
  note: BATT Control
  PV : Inport
  FC : Inport  Port=2
  SC : Inport  Port=3
  BATT : Inport  Port=4
  LOAD : Inport  Port=5
  Add : Sum  Inputs=+-
  Bus Selector : BusSelector  OutputSignals=Vfc,Ifc conv,Ifc,Ifc out
  Bus Selector1 : BusSelector  OutputSignals=Voltage (V),Current (A),current_command,Ibatt_output,SOC (%)
  Bus Selector2 : BusSelector  OutputSignals=V_PV,PV current demand,I_PV,Ibatt_output
  Bus Selector3 : BusSelector  OutputSignals=Vbus real,Vbus required,Pload required,Pload real
  Clock3 : Clock
  Constant : Constant  Value=IO_pv_conv_value
  Constant2 : Constant  Value=IO_fc_conv_value
  Constant20 : Constant  Value=270
  Constant3 : Constant  Value=cont_var_pv
  Constant4 : Constant  Value=IO_batt_conv_value
  Constant5 : Constant  Commented=on  Value=74
  Constant6 : Constant  Commented=on  Value=70
  Discrete PI Controller1 : Subsystem  Commented=on  DialogController=POWERSYS.PowerSysDialog  mask(Discrete PI Controller){Kp=1, Ki=10, Par_Limits=[100 -100], Init=0, Ts=1e-4}
      mask prompts: Kp "Proportional gain (Kp):"; Ki "Integral gain (Ki):"; Par_Limits "Output limits: [ Upper   Lower ]"; Init "Output initial value:"; Ts "Sample time:"
      mask help: This block implements a discrete PI controller.
      mask init:
      | UpperLimit=Par_Limits(1);
      | LowerLimit=Par_Limits(2);
      | power_initmask();
      mask Help: This block is part of a subset of blocks in the Extras library that does not have documentation associated with it, other than the block mask description.
      mask Display: disp('PI');
  Discrete PI Controller2 : Subsystem  DialogController=POWERSYS.PowerSysDialog  mask(Discrete PI Controller){Kp=10, Ki=100, Par_Limits=[100 -100], Init=0, Ts=1e-4}
      mask prompts: Kp "Proportional gain (Kp):"; Ki "Integral gain (Ki):"; Par_Limits "Output limits: [ Upper   Lower ]"; Init "Output initial value:"; Ts "Sample time:"
      mask help: This block implements a discrete PI controller.
      mask init:
      | UpperLimit=Par_Limits(1);
      | LowerLimit=Par_Limits(2);
      | power_initmask();
      mask Help: This block is part of a subset of blocks in the Extras library that does not have documentation associated with it, other than the block mask description.
      mask Display: disp('PI');
  Discrete PI Controller3 : Subsystem  Commented=on  DialogController=POWERSYS.PowerSysDialog  mask(Discrete PI Controller){Kp=10, Ki=1, Par_Limits=[100 -100], Init=0, Ts=1e-4}
      mask prompts: Kp "Proportional gain (Kp):"; Ki "Integral gain (Ki):"; Par_Limits "Output limits: [ Upper   Lower ]"; Init "Output initial value:"; Ts "Sample time:"
      mask help: This block implements a discrete PI controller.
      mask init:
      | UpperLimit=Par_Limits(1);
      | LowerLimit=Par_Limits(2);
      | power_initmask();
      mask Help: This block is part of a subset of blocks in the Extras library that does not have documentation associated with it, other than the block mask description.
      mask Display: disp('PI');
  Discrete PI Controller6 : Subsystem  Commented=on  DialogController=POWERSYS.PowerSysDialog  mask(Discrete PI Controller){Kp=10, Ki=10, Par_Limits=[40 0], Init=0, Ts=1e-4}
      mask prompts: Kp "Proportional gain (Kp):"; Ki "Integral gain (Ki):"; Par_Limits "Output limits: [ Upper   Lower ]"; Init "Output initial value:"; Ts "Sample time:"
      mask help: This block implements a discrete PI controller.
      mask init:
      | UpperLimit=Par_Limits(1);
      | LowerLimit=Par_Limits(2);
      | power_initmask();
      mask Help: This block is part of a subset of blocks in the Extras library that does not have documentation associated with it, other than the block mask description.
      mask Display: disp('PI');
  Discrete PI Controller7 : Subsystem  Commented=on  DialogController=POWERSYS.PowerSysDialog  mask(Discrete PI Controller){Kp=10, Ki=10, Par_Limits=[0 -40], Init=0, Ts=1e-4}
      mask prompts: Kp "Proportional gain (Kp):"; Ki "Integral gain (Ki):"; Par_Limits "Output limits: [ Upper   Lower ]"; Init "Output initial value:"; Ts "Sample time:"
      mask help: This block implements a discrete PI controller.
      mask init:
      | UpperLimit=Par_Limits(1);
      | LowerLimit=Par_Limits(2);
      | power_initmask();
      mask Help: This block is part of a subset of blocks in the Extras library that does not have documentation associated with it, other than the block mask description.
      mask Display: disp('PI');
  From108 : From  Commented=on  GotoTag=curr_batt_command_1
  From110 : From  Commented=on  GotoTag=curr_batt_command_2
  From16 : From  Commented=on  GotoTag=Ifc_boost
  From25 : From  Commented=on  GotoTag=curr_batt_command_3
  From26 : From  Commented=on  GotoTag=curr_batt_command_1
  From30 : From  Commented=on  GotoTag=Vbus_required
  MATLAB Function : MATLAB Function  TreatAsAtomicUnit=on
  MATLAB Function1 : MATLAB Function  TreatAsAtomicUnit=on
  Mux2 : Mux  Inputs=2
  PV - FC - control : MATLAB Function  TreatAsAtomicUnit=on
  S-Function2 : S-Function  FunctionName=EEMS  SFunctionDeploymentMode=off  EnableBusSupport=off
  Saturation4 : Saturate  UpperLimit=8800  LowerLimit=850
  Saturation7 : Saturate  UpperLimit=3400  LowerLimit=-1500
  Saturation8 : Saturate  UpperLimit=2  LowerLimit=-2
  Selector7 : Selector  InputPortWidth=2  IndexOptions=Index vector (dialog)  Indices=1  OutputSizes=1
  Selector8 : Selector  InputPortWidth=2  IndexOptions=Index vector (dialog)  Indices=2  OutputSizes=1
  Sum : Sum  Inputs=|+-
  Sum1 : Sum  Commented=on  Inputs=|+-
  Sum{2..5,8..9} (6 alike) : Sum  Inputs=|++
  Sum6 : Sum  Commented=on  Inputs=|+-
  Sum7 : Sum  Commented=on  Inputs=|+-
  Zero-Order Hold : ZeroOrderHold  SampleTime=1e-4
  Zero-Order Hold1 : ZeroOrderHold  SampleTime=200e-3
  Vbatt_conv : Outport
  Ibatt_conv : Outport  Port=2
  batt converter mode : Outport  Port=3
  I/O batt conv : Outport  Port=4
  Vfc_conv : Outport  Port=5
  Ifc_conv : Outport  Port=6
  I/O fc conv : Outport  Port=7
  Vpv_conv : Outport  Port=8
  Ipv_conv : Outport  Port=9
  I/O pv conv : Outport  Port=10
  PV control mode : Outport  Port=11
  tag scope: Vdcref=global
  wires:
  [Ipv_out] -> PV - FC - control/11(Ipvout)
  Sum1/1 -> Sum2/2
  PV - FC - control/7(Control_pv) -> [Control_pv]
  [Vbus_required] -> PV - FC - control/2(Vdc_command)
  MATLAB Function/4(IO_batt_conv) -> [IO_batt_conv]
  Constant3/1 -> PV - FC - control/16(Control_pv_choose_var)
  [Vbatt_conv] -> Vbatt_conv/1
  [Vbus_real] -> PV - FC - control/12(Vdc_real)
  [Pload] -> MATLAB Function/8(Pload)
  Zero-Order Hold/1 -> PV - FC - control/1(Time)  "time"
  [Ipv] -> PV - FC - control/9(Ipv_in)
  Sum8/1 -> Sum2/1  "Batt current command"
  [Vpv] -> PV - FC - control/7(Vpv)
  LOAD/1 -> Bus Selector3/1
  Clock3/1 -> Zero-Order Hold/1  "time"
  [Control_pv] -> PV control mode/1
  [Ipv_out] -> MATLAB Function/7(Ipv_out)
  Bus Selector/3 -> [Ifc]  "<Ifc>"
  [IO_batt_conv] -> I/O batt conv/1
  Bus Selector3/3 -> [Pload]  "<Pload required>"
  PV - FC - control/4(Ipv) -> [Ipv_boost]  "PV current demand"
  Bus Selector2/4 -> [Ipv_out]  "<Ibatt_output>"
  [Ifc_boost] -> Sum4/1
  [Vbus_required] -> MATLAB Function/10(Vdc_wanted)
  [BATT_SOC] -> PV - FC - control/17(BATT_SOC)
  PV/1 -> Bus Selector2/1
  [curr_batt_command_3] -> Discrete PI Controller2/1(Error)  "Batt current command 3"
  From110/1 -> Discrete PI Controller3/1(Error)  "Batt current command 3"
  [Vbus_required] -> MATLAB Function1/3(Vbus_required)
  Bus Selector1/3 -> [Ibatt_command_pre]  "<current_command>"
  PV - FC - control/3(IO_fc_conv) -> [IO_fc_boost]
  [Ifc_out] -> MATLAB Function/4(Ifc_out)
  [Vpv_conv] -> Vpv_conv/1
  Bus Selector1/2 -> [Ibatt]  "<Current (A)>"
  MATLAB Function1/3(V_batt_conv) -> [Vbatt_conv]
  [Ifc_boost] -> MATLAB Function/13(Ifc_boost)
  Bus Selector/2 -> [Ifc_boost_prev]  "<Ifc conv>"
  Bus Selector3/4 -> [Pload_real]  "<Pload real>"
  Discrete PI Controller3/1(Out) -> Sum9/2
  [Ifc] -> PV - FC - control/4(Ifc_in)
  Discrete PI Controller6/1(Out) -> Sum4/2
  [Vbatt] -> MATLAB Function/1(Vbatt)
  PV - FC - control/6(IO_pv_conv) -> [IO_pv_boost]
  Discrete PI Controller2/1(Out) -> Sum8/2
  Bus Selector1/5 -> [BATT_SOC]  "<SOC (%)>"
  Bus Selector1/4 -> [Ibatt_out]  "<Ibatt_output>"
  [Vbatt] -> PV - FC - control/5(Vbatt)
  [Ipv_boost] -> Ipv_conv/1
  Sum7/1 -> Discrete PI Controller6/1(Error)
  Bus Selector3/2 -> [Vbus_required]  "<Vbus required>"
  Bus Selector3/1 -> [Vbus_real]  "<Vbus real>"
  Bus Selector2/2 -> [Ipv_boost_prev]  "<PV current demand>"
  FC/1 -> Bus Selector/1
  PV - FC - control/2(Vfc_conv) -> [Vfc_conv]
  Bus Selector/4 -> [Ifc_out]  "<Ifc out>"
  PV - FC - control/1(Ifc) -> [Ifc_boost]
  [BATT_SOC] -> PV - FC - control/10(SOC)
  [Vfc] -> PV - FC - control/3(Vfc)
  [Pload] -> PV - FC - control/8(Pload)
  Sum6/1 -> Discrete PI Controller7/1(Error)
  From26/1 -> Sum1/1  "Batt current command 1"
  [Pload_real] -> MATLAB Function/11(Pout)
  PV - FC - control/5(Vpv_conv) -> [Vpv_conv]
  MATLAB Function1/2(current_command) -> [I_batt_charge]
  [Ibatt_out] -> MATLAB Function/3(Ibatt_out)
  Constant6/1 -> Sum6/1
  Sum4/1 -> Sum3/1
  SC/1 -> [SC_SOC]
  [Ipv] -> MATLAB Function/6(Ipv)
  Bus Selector2/1 -> [Vpv]  "<V_PV>"
  Constant2/1 -> PV - FC - control/15(IO_fc_conv_value)
  [Pload] -> MATLAB Function1/2(Pload)
  MATLAB Function/1(Ibatt_1) -> [curr_batt_command_1]
  Constant5/1 -> Sum7/1
  Constant4/1 -> MATLAB Function/12(IO_batt_conv_value)
  MATLAB Function/2(Ibatt_2) -> [curr_batt_command_2]
  [IO_fc_boost] -> I/O fc conv/1
  [Ibatt] -> MATLAB Function/2(Ibatt)
  From108/1 -> Discrete PI Controller1/1(Error)  "Batt current command 1"
  [IO_pv_boost] -> I/O pv conv/1
  Bus Selector2/3 -> [Ipv]  "<I_PV>"
  [Vfc] -> MATLAB Function/14(Vfc)
  MATLAB Function/3(Ibatt_3) -> [curr_batt_command_3]
  From25/1 -> Sum1/2  "Batt current command 3"
  BATT/1 -> Bus Selector1/1
  Sum3/1 -> Ifc_conv/1
  [Vfc_conv] -> Vfc_conv/1
  Sum2/1 -> MATLAB Function1/1(current_comm)  "Batt current command"
  Bus Selector/1 -> [Vfc]  "<Vfc>"
  [Pload_real] -> PV - FC - control/13(Pout_real)
  [Ibatt] -> PV - FC - control/6(Ibatt_in)
  [Vpv] -> MATLAB Function/5(Vpv)
  [Vbus_real] -> MATLAB Function/9(Vdc)
  Discrete PI Controller7/1(Out) -> Sum3/2
  Bus Selector1/1 -> [Vbatt]  "<Voltage (V)>"
  Sum9/1 -> Sum8/1
  [Converter] -> batt converter mode/1
  MATLAB Function1/1(conv) -> [Converter]
  Constant/1 -> PV - FC - control/14(IO_pv_conv_value)
  [I_batt_charge] -> Ibatt_conv/1
  From30/1 -> Sum6/2, Sum7/2
  Discrete PI Controller1/1(Out) -> Sum9/1
  Selector7/1 -> Saturation7/1
  Saturation7/1 -> Add/2
  ? -> Add/1
  Saturation4/1 -> ?
  Selector8/1 -> Saturation8/1
  Add/1 -> Saturation4/1
  Saturation8/1 -> Sum5/2
  S-Function2/1 -> Selector7/1, Selector8/1
  [Vdc] -> Zero-Order Hold1/1, Sum/2
  Constant20/1 -> Sum5/1
  ? -> Mux2/1
  Mux2/1 -> S-Function2/1
  Zero-Order Hold1/1 -> Mux2/2
  Sum5/1 -> [Vdcref], Sum/1
  PV - FC - control/8(DV) -> [DV]
  [DV] -> MATLAB Function1/4(DV)
